simulink model "convolutionalcode_11"  (R2018a)
settings: Solver=VariableStepAuto  StartTime=0.0  StopTime=10.0  RelTol=1e-3
values from neighbouring files (symbols this model uses):
  BitRate = 100000    [convolutionalcode_1111.m]
  Lc = 7    [convolutionalcode_1111.m]
libraries: commcnvcod2 x3, commdigbbndpm3 x2, commsink2 x2, commchan3 x1, commrandsrc3 x1
settings Model: Creator=sdf  LastModifiedBy=sdf

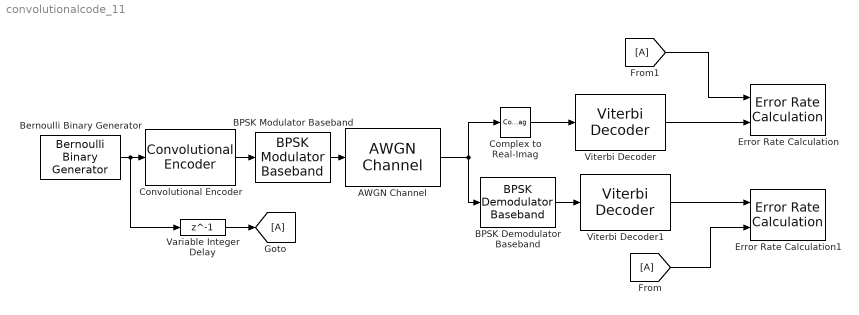
== system convolutionalcode_11 ==
  AWGN Channel : commchan3/AWGN Channel  InputProcessing=Columns as channels (frame based)  seed=67  noiseMode="Signal to noise ratio  (Eb/No)"  EbNodB=SNR  EsNodB=10  SNRdB=10  bitsPerSym=1  Ps=1  Tsym=1/BitRate  variance=1
  BPSK Demodulator Baseband : commdigbbndpm3/BPSK Demodulator Baseband  DecType=Hard decision  VarSource=Dialog  Variance=1  Ph=0  outDtype=Inherit via internal rule  derotateFactorWordLen=16  derotateFactorDataTypeStr=Inherit: Same word length as input  derotateFactorLastDataTypeStr=Inherit: Same word length as input
  BPSK Modulator Baseband : commdigbbndpm3/BPSK Modulator Baseband  Ph=0  outDtype=double  outWordLen=16  outUDDataType=sfix(16)  outFracLenMode=Best precision  outFracLen=15  outDataTypeStr=double  outLastDataTypeStr=double
  Bernoulli Binary Generator : commrandsrc3/Bernoulli Binary Generator  ProbabilityOfZero=0.5  SeedSource=Parameter  Seed=61  SampleTime=1/BitRate  SamplesPerFrame=BitRate  OutputDataType=double  SimulateUsing=Interpreted execution
  Complex to Real-Imag : ComplexToRealImag  Output=Real
  Convolutional Encoder : commcnvcod2/Convolutional Encoder  trellis=poly2trellis(Lc, [171 133])  opMode=Continuous  DelayedResetAction=off  hasIniStPort=off  hasFinStPort=off  usePuncVector=off  punctureVector=[1; 1; 0; 1; 0; 1]  reset=Unused parameter value
      settings: SourceProductName=Communications System Toolbox  SourceProductBaseCode=CM
  Error Rate Calculation : commsink2/Error Rate Calculation  N=0  st_delay=0  cp_mode=Entire frame  subframe=[]  PMode=Workspace  WsName=BER2  RsMode2=off  stop=off  numErr=100  maxBits=1e6
  Error Rate Calculation1 : commsink2/Error Rate Calculation  N=0  st_delay=0  cp_mode=Entire frame  subframe=[]  PMode=Workspace  WsName=BER1  RsMode2=off  stop=off  numErr=100  maxBits=1e6
  Variable Integer Delay : Delay  DelayLength=1  InputProcessing=Columns as channels (frame based)
  Viterbi Decoder : commcnvcod2/Viterbi Decoder  trellis=poly2trellis(Lc, [171 133])  isPunctured=off  punctureVector=[1; 1; 0; 1; 0; 1]  erasures=off  dectype=Unquantized  nsdecb=4  runSigValErrCheck=off  tbdepth=6*Lc  opmode=Continuous  reset=off  delayedResetAction=off  smWordLength=16  outDataType=Inherit via internal rule
      settings: SourceProductName=Communications System Toolbox  SourceProductBaseCode=CM
  Viterbi Decoder1 : commcnvcod2/Viterbi Decoder  trellis=poly2trellis(Lc, [171 133])  isPunctured=off  punctureVector=[1; 1; 0; 1; 0; 1]  erasures=off  dectype=Hard decision  nsdecb=4  runSigValErrCheck=off  tbdepth=6*Lc  opmode=Continuous  reset=off  delayedResetAction=off  smWordLength=16  outDataType=Inherit via internal rule
      settings: SourceProductName=Communications System Toolbox  SourceProductBaseCode=CM
  wires:
  Bernoulli Binary Generator/1 -> Variable Integer Delay/1, Convolutional Encoder/1
  Convolutional Encoder/1 -> BPSK Modulator Baseband/1
  Variable Integer Delay/1 -> [A]
  BPSK Modulator Baseband/1 -> AWGN Channel/1
  AWGN Channel/1 -> Complex to Real-Imag/1, BPSK Demodulator Baseband/1
  Complex to Real-Imag/1 -> Viterbi Decoder/1
  BPSK Demodulator Baseband/1 -> Viterbi Decoder1/1
  Viterbi Decoder/1 -> Error Rate Calculation/2
  [A] -> Error Rate Calculation/1
  Viterbi Decoder1/1 -> Error Rate Calculation1/1
  [A] -> Error Rate Calculation1/2
